simulink model "simscapeTest"  (R2013a)
settings: Solver=ode45  StartTime=0.0  StopTime=10.0  RelTol=1e-3
undefined symbols (not defined in the file or in its folder): R1, R2
libraries: fl_lib x4, elec_lib x1, nesl_utility x1
settings Model: Creator=mainster  LastModifiedBy=mainster

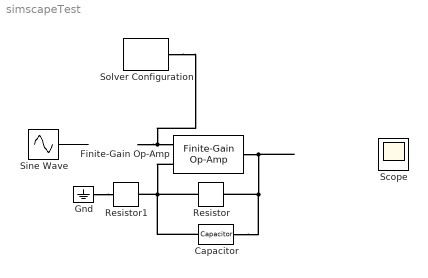
== system simscapeTest ==
  Capacitor : fl_lib/Electrical/Electrical Elements/Capacitor  c=C F  v0=0 V  r=1e-6 Ohm  g=0 1/Ohm  i_Log=off  v_Log=off  vc_Log=off  LocalVarNames=|i|v|vc  LocalVarDescs=|i|v|Internal variable for voltage across capacitor term  LocalVarLogging=[0 0 0]
      settings: AttributesFormatString=%<c>
  Finite-Gain Op-Amp : elec_lib/Integrated Circuits/Finite-Gain Op-Amp  A=1000  Rin=1e+6 Ohm  Rout=100 Ohm  Vmin=-15 V  Vmax=15 V  LocalVarLogging=[]
  Gnd : fl_lib/Electrical/Electrical Elements/Electrical Reference  i_Log=off  LocalVarNames=|i  LocalVarDescs=|i  LocalVarLogging=0
  Resistor : fl_lib/Electrical/Electrical Elements/Resistor  R=R2 Ohm  i_Log=off  v_Log=off  LocalVarNames=|i|v  LocalVarDescs=|i|v  LocalVarLogging=[0 0]
      settings: AttributesFormatString=%<R>
  Resistor1 : fl_lib/Electrical/Electrical Elements/Resistor  R=R1 Ohm  i_Log=off  v_Log=off  LocalVarNames=|i|v  LocalVarDescs=|i|v  LocalVarLogging=[0 0]
      settings: AttributesFormatString=%<R>
  Scope : Scope
  Sine Wave : Sin  SampleTime=0
  Solver Configuration : nesl_utility/Solver Configuration  PhysicalDomain=network_engine_domain  SubClassName=solver  LeftPortType=input  RightPortType=generic  Accelerate=off  Tones=[]  Harmonics=[]  SimulateNoise=off  Profile=off  UseLocalSampling=off  EnableSwitchedLinearOptims=on  FrequencyDomain=off  UseCCode=off  UseNewInitialization=off  DoDC=off  ResidualTolerance=1e-09  UseLocalSolver=off  LocalSolverChoice=NE_BACKWARD_EULER_ADVANCER  LocalSolverSampleTime=0.001  DoFixedCost=off  MaxNonlinIter=3  MaxModeIter=2  LinearAlgebra=Sparse  DelaysMemoryBudget=1024
  wires:
  ? -> Scope/1
  Sine Wave/1 -> ?
  connections:
  Resistor/RConn1 -- Finite-Gain Op-Amp/RConn1 -- Capacitor/RConn1
  Resistor/LConn1 -- Resistor1/RConn1 -- Capacitor/LConn1 -- Finite-Gain Op-Amp/LConn2
  Gnd/LConn1 -- Resistor1/LConn1
  Solver Configuration/RConn1 -- Finite-Gain Op-Amp/LConn1
